simulink model "drone_impl"  (R2023a)
settings: configuration reference "Configuration" (kept outside this file)
settings Model: DataDictionary=data.sldd  Creator=tmiura  LastModifiedBy=tmiura
settings ConfigSetRef: SourceName=Configuration

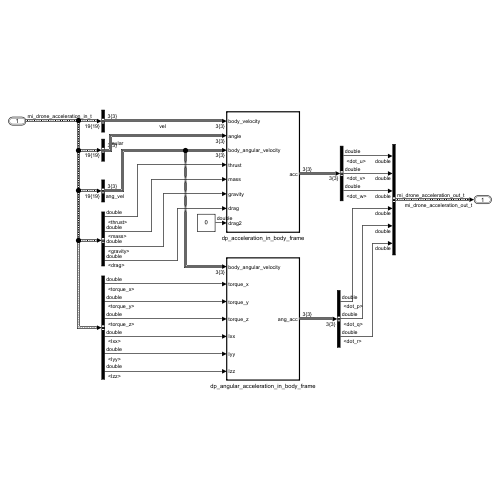
[thumbnail: Simulink's stored preview of the top-level diagram]
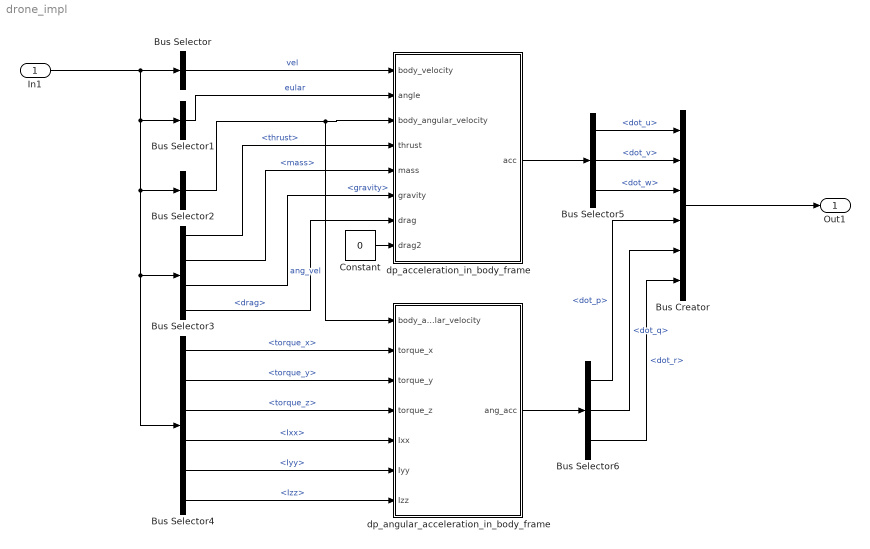
== system drone_impl ==
  In1 : Inport  OutDataTypeStr=Bus: mi_drone_acceleration_in_t  BusOutputAsStruct=on
  Bus Creator : BusCreator  Inputs=6  OutDataTypeStr=Bus: mi_drone_acceleration_out_t  NonVirtualBus=on
      settings: InheritFromInputs=off
  Bus Selector : BusSelector  OutputSignals=u,v,w  OutputAsBus=on
  Bus Selector1 : BusSelector  OutputSignals=phi,theta,psi  OutputAsBus=on
  Bus Selector2 : BusSelector  OutputSignals=p,q,r  OutputAsBus=on
  Bus Selector3 : BusSelector  OutputSignals=thrust,mass,gravity,drag
  Bus Selector4 : BusSelector  OutputSignals=torque_x,torque_y,torque_z,Ixx,Iyy,Izz
  Bus Selector5 : BusSelector  OutputSignals=dot_u,dot_v,dot_w
  Bus Selector6 : BusSelector  OutputSignals=dot_p,dot_q,dot_r
  Constant : Constant  Value=0
  dp_acceleration_in_body_frame : Subsystem  TreatAsAtomicUnit=on
      settings: RTWFcnNameOpts=Use subsystem name  FunctionInterfaceSpec=Allow arguments (Optimized)
  dp_angular_acceleration_in_body_frame : Subsystem  TreatAsAtomicUnit=on
      settings: RTWFcnNameOpts=Use subsystem name  FunctionInterfaceSpec=Allow arguments (Optimized)
  Out1 : Outport  OutDataTypeStr=Bus: mi_drone_acceleration_out_t  BusOutputAsStruct=on
  wires:
  In1/1 -> Bus Selector4/1, Bus Selector3/1, Bus Selector2/1, Bus Selector1/1, Bus Selector/1
  Bus Creator/1 -> Out1/1
  Bus Selector/1 -> dp_acceleration_in_body_frame/1(body_velocity)  "vel"
  Bus Selector1/1 -> dp_acceleration_in_body_frame/2(angle)  "eular"
  Bus Selector2/1 -> dp_acceleration_in_body_frame/3(body_angular_velocity), dp_angular_acceleration_in_body_frame/1(body_angular_velocity)  "ang_vel"
  Bus Selector3/1 -> dp_acceleration_in_body_frame/4(thrust)  "<thrust>"
  Bus Selector3/2 -> dp_acceleration_in_body_frame/5(mass)  "<mass>"
  Bus Selector3/3 -> dp_acceleration_in_body_frame/6(gravity)  "<gravity>"
  Bus Selector3/4 -> dp_acceleration_in_body_frame/7(drag)  "<drag>"
  Bus Selector4/1 -> dp_angular_acceleration_in_body_frame/2(torque_x)  "<torque_x>"
  Bus Selector4/2 -> dp_angular_acceleration_in_body_frame/3(torque_y)  "<torque_y>"
  Bus Selector4/3 -> dp_angular_acceleration_in_body_frame/4(torque_z)  "<torque_z>"
  Bus Selector4/4 -> dp_angular_acceleration_in_body_frame/5(Ixx)  "<Ixx>"
  Bus Selector4/5 -> dp_angular_acceleration_in_body_frame/6(Iyy)  "<Iyy>"
  Bus Selector4/6 -> dp_angular_acceleration_in_body_frame/7(Izz)  "<Izz>"
  Constant/1 -> dp_acceleration_in_body_frame/8(drag2)
  dp_acceleration_in_body_frame/1(acc) -> Bus Selector5/1
  dp_angular_acceleration_in_body_frame/1(ang_acc) -> Bus Selector6/1
  Bus Selector5/1 -> Bus Creator/1  "<dot_u>"
  Bus Selector5/2 -> Bus Creator/2  "<dot_v>"
  Bus Selector5/3 -> Bus Creator/3  "<dot_w>"
  Bus Selector6/1 -> Bus Creator/4  "<dot_p>"
  Bus Selector6/2 -> Bus Creator/5  "<dot_q>"
  Bus Selector6/3 -> Bus Creator/6  "<dot_r>"

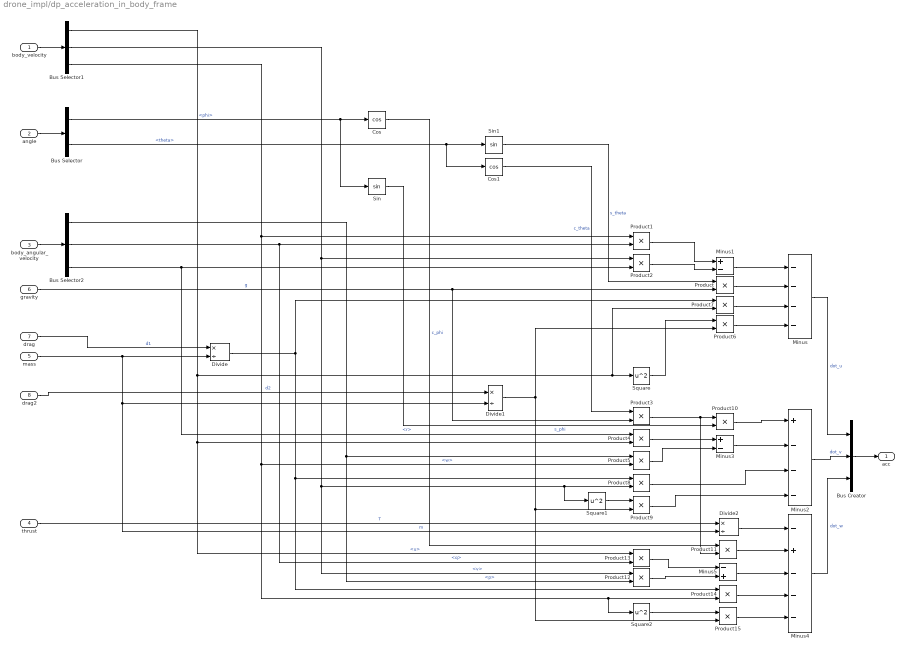
== system drone_impl/dp_acceleration_in_body_frame ==
  body_velocity : Inport
  angle : Inport  Port=2
  body_angular_velocity : Inport  Port=3
  thrust : Inport  Port=4
  mass : Inport  Port=5
  gravity : Inport  Port=6
  drag : Inport  Port=7
  drag2 : Inport  Port=8
  Bus Creator : BusCreator  Inputs=3
  Bus Selector : BusSelector  OutputSignals=phi,theta
  Bus Selector1 : BusSelector  OutputSignals=u,v,w
  Bus Selector2 : BusSelector  OutputSignals=p,q,r
  Cos : Trigonometry  Operator=cos
  Cos1 : Trigonometry  Operator=cos
  Divide : Product  Inputs=*/
  Divide1 : Product  Inputs=*/
  Divide2 : Product  Inputs=*/
  Minus : Sum  Inputs=----
  Minus1 : Sum  Inputs=+-
  Minus2 : Sum  Inputs=+---
  Minus3 : Sum  Inputs=+-
  Minus4 : Sum  Inputs=-+---
  Minus5 : Sum  Inputs=-+
  Product{,1..15} (16 alike) : Product
  Sin : Trigonometry
  Sin1 : Trigonometry
  Square : Math  Operator=square
  Square1 : Math  Operator=square
  Square2 : Math  Operator=square
  acc : Outport
  wires:
  body_velocity/1 -> Bus Selector1/1
  angle/1 -> Bus Selector/1
  Bus Selector/1 -> Cos/1, Sin/1  "<phi>"
  Sin/1 -> Product10/2  "s_phi"
  Cos/1 -> Product11/1  "c_phi"
  Cos1/1 -> Product3/1  "c_theta"
  Bus Selector/2 -> Cos1/1, Sin1/1  "<theta>"
  body_angular_velocity/1 -> Bus Selector2/1
  thrust/1 -> Divide2/1  "T"
  mass/1 -> Divide2/2, Divide1/2, Divide/2  "m"
  gravity/1 -> Product3/2, Product/2  "g"
  drag/1 -> Divide/1  "d1"
  drag2/1 -> Divide1/1  "d2"
  Sin1/1 -> Product/1  "s_theta"
  Bus Selector1/1 -> Product4/2, Product13/1, Product7/2, Square/1  "<u>"
  Bus Selector1/2 -> Product12/1, Square1/1, Product8/2, Product2/1  "<v>"
  Bus Selector1/3 -> Square2/1, Product14/2, Product5/2, Product1/1  "<w>"
  Bus Selector2/1 -> Product12/2, Product5/1  "<p>"
  Bus Selector2/2 -> Product13/2, Product1/2  "<q>"
  Bus Selector2/3 -> Product4/1, Product2/2  "<r>"
  Product1/1 -> Minus1/1
  Product2/1 -> Minus1/2
  Product/1 -> Minus/2
  Minus1/1 -> Minus/1
  Divide1/1 -> Product15/2, Product9/2, Product6/2
  Minus/1 -> Bus Creator/1  "dot_u"
  Product3/1 -> Product11/2, Product10/1
  Product4/1 -> Minus3/1
  Product5/1 -> Minus3/2
  Minus3/1 -> Minus2/2
  Square/1 -> Product6/1
  Product6/1 -> Minus/4
  Divide/1 -> Product14/1, Product8/1, Product7/1
  Product7/1 -> Minus/3
  Square1/1 -> Product9/1
  Product8/1 -> Minus2/3
  Product9/1 -> Minus2/4
  Minus2/1 -> Bus Creator/2  "dot_v"
  Divide2/1 -> Minus4/1
  Product10/1 -> Minus2/1
  Product11/1 -> Minus4/2
  Product13/1 -> Minus5/1
  Product12/1 -> Minus5/2
  Minus5/1 -> Minus4/3
  Minus4/1 -> Bus Creator/3  "dot_w"
  Product14/1 -> Minus4/4
  Square2/1 -> Product15/1
  Product15/1 -> Minus4/5
  Bus Creator/1 -> acc/1

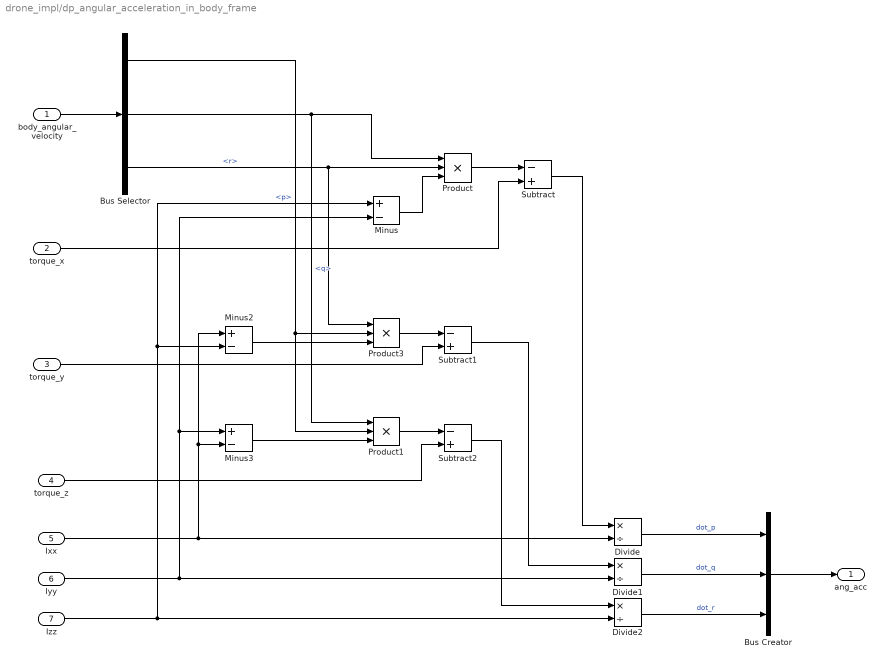
== system drone_impl/dp_angular_acceleration_in_body_frame ==
  body_angular_velocity : Inport
  torque_x : Inport  Port=2
  torque_y : Inport  Port=3
  torque_z : Inport  Port=4
  Ixx : Inport  Port=5
  Iyy : Inport  Port=6
  Izz : Inport  Port=7
  Bus Creator : BusCreator  Inputs=3
  Bus Selector : BusSelector  OutputSignals=p,q,r
  Divide : Product  Inputs=*/
  Divide1 : Product  Inputs=*/
  Divide2 : Product  Inputs=*/
  Minus : Sum  Inputs=+-
  Minus2 : Sum  Inputs=+-
  Minus3 : Sum  Inputs=+-
  Product : Product  Inputs=3
  Product1 : Product  Inputs=3
  Product3 : Product  Inputs=3
  Subtract : Sum  Inputs=-+
  Subtract1 : Sum  Inputs=-+
  Subtract2 : Sum  Inputs=-+
  ang_acc : Outport
  wires:
  body_angular_velocity/1 -> Bus Selector/1
  Bus Selector/1 -> Product1/2, Product3/2  "<p>"
  Bus Selector/2 -> Product1/1, Product/1  "<q>"
  Bus Selector/3 -> Product3/1, Product/2  "<r>"
  Subtract/1 -> Divide/1
  Ixx/1 -> Divide/2, Minus3/2, Minus2/1
  Divide/1 -> Bus Creator/1  "dot_p"
  torque_x/1 -> Subtract/2
  Izz/1 -> Minus2/2, Minus/1, Divide2/2
  Iyy/1 -> Divide1/2, Minus3/1, Minus/2
  Minus/1 -> Product/3
  Product/1 -> Subtract/1
  Bus Creator/1 -> ang_acc/1
  torque_y/1 -> Subtract1/2
  Subtract1/1 -> Divide1/1
  Product3/1 -> Subtract1/1
  Minus2/1 -> Product3/3
  Divide1/1 -> Bus Creator/2  "dot_q"
  Divide2/1 -> Bus Creator/3  "dot_r"
  Subtract2/1 -> Divide2/1
  Product1/1 -> Subtract2/1
  Minus3/1 -> Product1/3
  torque_z/1 -> Subtract2/2
